simulink model "integr_1"  (Simulink 3.00)
settings: Solver=ode45  SolverMode=SingleTasking  StartTime=0.0  StopTime=30.0  RelTol=1e-3  AbsTol=1e-6
libraries: simulink3 x1
settings Model: LimitMaxRows=on

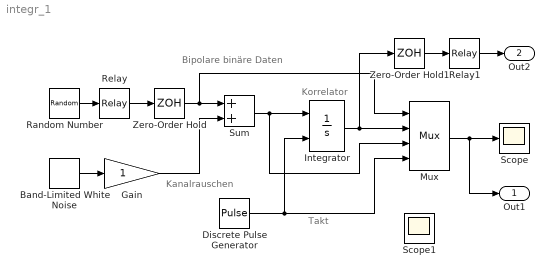
== system integr_1 ==
  note: Bipolare binäre Daten
  note: Kanalrauschen
  note: Takt
  note: Korrelator
  Band-Limited White Noise : simulink3/Sources/Band-Limited White Noise  Cov=[0.1]  Ts=0.1  seed=[23341]
  Discrete Pulse Generator : DiscretePulseGenerator  Amplitude=1  Period=10  PulseWidth=5  PhaseDelay=0  SampleTime=0.1
  Gain : Gain  Gain=1  SaturateOnIntegerOverflow=on
  Integrator : Integrator  ExternalReset=rising  InitialConditionSource=internal  InitialCondition=0  LimitOutput=off  UpperSaturationLimit=inf  LowerSaturationLimit=-inf  ShowSaturationPort=off  ShowStatePort=off  AbsoluteTolerance=auto
  Mux : Mux  Inputs=4
      settings: DisplayOption=none
  Random Number : RandomNumber  Mean=0  Variance=1  Seed=0  SampleTime=0
  Relay : Relay  OnSwitchValue=eps  OffSwitchValue=eps  OnOutputValue=1  OffOutputValue=-1
  Relay1 : Relay  OnSwitchValue=eps  OffSwitchValue=eps  OnOutputValue=1  OffOutputValue=-1
  Scope : Scope
      settings: TickLabels=on  TimeRange=auto  YMin=-5  YMax=5  SaveToWorkspace=off  SaveName=ScopeData  DataFormat=Matrix
  Scope1 : Scope
      settings: Floating=on  TickLabels=on  TimeRange=auto  YMin=-2  YMax=2  SaveToWorkspace=off  SaveName=ScopeData  DataFormat=Matrix
  Sum : Sum  Inputs=++  SaturateOnIntegerOverflow=on
  Zero-Order Hold : ZeroOrderHold  SampleTime=1
  Zero-Order Hold1 : ZeroOrderHold  SampleTime=[1 0.8]
  Out1 : Outport  Port=1
  Out2 : Outport  Port=2
  wires:
  Random Number/1 -> Relay/1
  Relay/1 -> Zero-Order Hold/1
  Band-Limited White Noise/1 -> Gain/1
  Zero-Order Hold/1 -> Sum/1, Mux/1
  Discrete Pulse Generator/1 -> Integrator/2, Mux/4
  Integrator/1 -> Mux/2, Zero-Order Hold1/1
  Mux/1 -> Scope/1, Out1/1
  Zero-Order Hold1/1 -> Relay1/1
  Relay1/1 -> Out2/1
  Gain/1 -> Sum/2
  Sum/1 -> Integrator/1, Mux/3
